simulink model "VCUHVACT"  (R2024b)
settings: Solver=FixedStepDiscrete  StartTime=0.0  StopTime=10.0  FixedStep=0.1  RelTol=1e-3
libraries: simulink x3
settings Model: Creator=32032  LastModifiedBy=32032
settings DataIOCC: SaveFormat=StructureWithTime
settings OptimizationCC: DefaultParameterBehavior=Inlined  EnhancedBackFolding=on  PassReuseOutputArgsAs=Individual arguments  ZeroExternalMemoryAtStartup=off  ZeroInternalMemoryAtStartup=off  OptimizeBlockOrder=speed  DifferentSizesBufferReuse=on  OptimizationCustomize=off  EfficientTunableParamExpr=on
settings DebuggingCC: ParameterTunabilityLossMsg=error
settings ModelReferenceCC: ModelReferenceNumInstancesAllowed=Single
settings SFSimCC: MATLABDynamicMemAlloc=off
settings RTWCC: Description=AUTOSAR  SystemTargetFile=autosar.tlc  GenCodeOnly=on  TemplateMakefile=ert_default_tmf  DataTypeReplacement=CDataTypesFixedWidth
settings CodeAppCC: ForceParamTrailComments=on  IgnoreCustomStorageClasses=off  OperatorAnnotations=on  SimulinkDataObjDesc=on  SFDataObjDesc=on  InsertBlockDesc=on
settings STFCustomTargetCC: TargetLangStandard=C99 (ISO)  MultiwordLength=256  ParMdlRefBuildCompliant=on  CompOptLevelCompliant=on  IncludeMdlTerminateFcn=off  CombineOutputUpdateFcns=on  SuppressErrorStatus=on  ERTCustomFileBanners=on  SupportNonFinite=off  SupportComplex=off  SupportContinuousTime=off  SupportNonInlinedSFcns=off  RemoveResetFunc=on  MATLABClassNameForMDSCustomization=Simulink.SoftwareTarget.ERTCustomization  AutosarCompliant=on  UseToolchainInfoCompliant=on  LookupTableObjectStructAxisOrder=2,1,3,4,...  LUTObjectStructOrderEvenSpacing=Size,Table,Breakpoints  SystemTargetFile=autosar.tlc
settings ERTTargetCC: TargetLangStandard=C99 (ISO)  ConcurrentExecutionCompliant=off  IncludeMdlTerminateFcn=off  SuppressErrorStatus=on  SupportNonFinite=off  SupportComplex=off  ModelStepFunctionPrototypeControlCompliant=off  CPPClassGenCompliant=off  AutosarCompliant=on  LookupTableObjectStructAxisOrder=2,1,3,4,...  LUTObjectStructOrderEvenSpacing=Size,Table,Breakpoints  ERTCustomFileTemplate=example_file_process.tlc  BooleanTrueId=TRUE  BooleanFalseId=FALSE

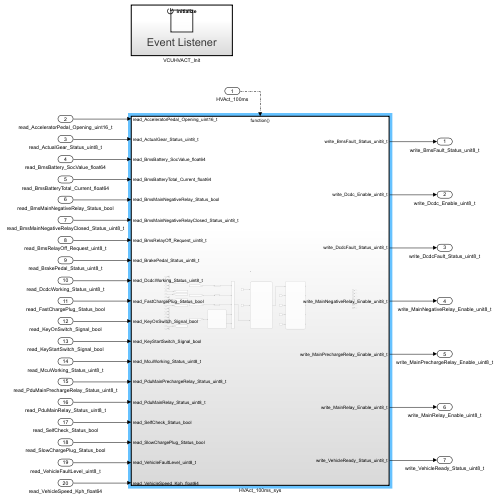
[thumbnail: Simulink's stored preview of the top-level diagram]
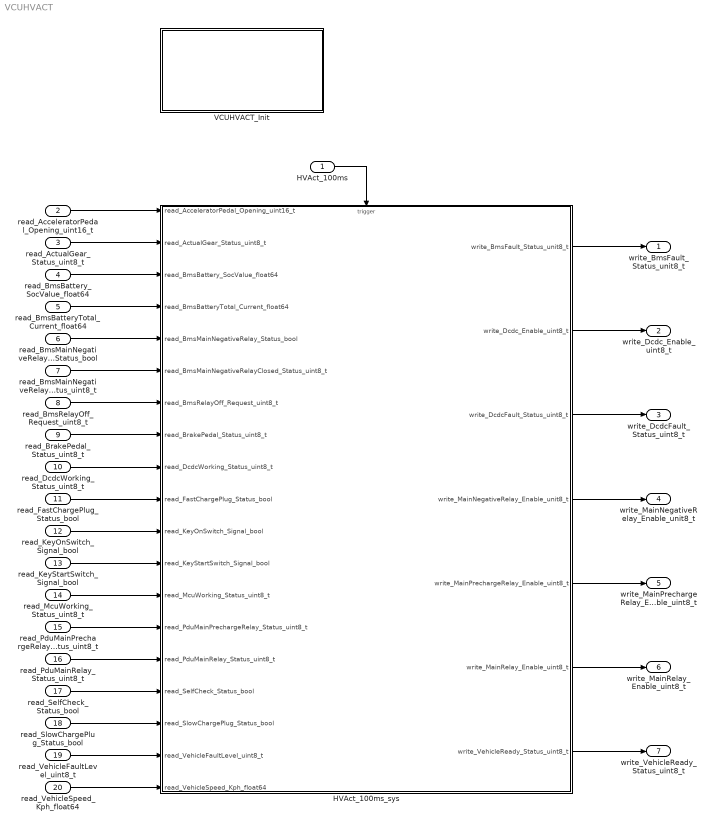
== system VCUHVACT ==
  HVAct_100ms : Inport  SampleTime=0.1  OutputFunctionCall=on
  read_AcceleratorPedal_Opening_uint16_t : Inport  Port=2  OutDataTypeStr=uint16  PortDimensions=1
  read_ActualGear_Status_uint8_t : Inport  Port=3  OutDataTypeStr=uint8  PortDimensions=1
  read_BmsBattery_SocValue_float64 : Inport  Port=4  OutDataTypeStr=double  PortDimensions=1
  read_BmsBatteryTotal_Current_float64 : Inport  Port=5  OutDataTypeStr=double  PortDimensions=1
  read_BmsMainNegativeRelay_Status_bool : Inport  Port=6  OutDataTypeStr=boolean  PortDimensions=1
  read_BmsMainNegativeRelayClosed_Status_uint8_t : Inport  Port=7  OutDataTypeStr=uint8  PortDimensions=1
  read_BmsRelayOff_Request_uint8_t : Inport  Port=8  OutDataTypeStr=uint8  PortDimensions=1
  read_BrakePedal_Status_uint8_t : Inport  Port=9  OutDataTypeStr=uint8  PortDimensions=1
  read_DcdcWorking_Status_uint8_t : Inport  Port=10  OutDataTypeStr=uint8  PortDimensions=1
  read_FastChargePlug_Status_bool : Inport  Port=11  OutDataTypeStr=boolean  PortDimensions=1
  read_KeyOnSwitch_Signal_bool : Inport  Port=12  OutDataTypeStr=boolean  PortDimensions=1
  read_KeyStartSwitch_Signal_bool : Inport  Port=13  OutDataTypeStr=boolean  PortDimensions=1
  read_McuWorking_Status_uint8_t : Inport  Port=14  OutDataTypeStr=uint8  PortDimensions=1
  read_PduMainPrechargeRelay_Status_uint8_t : Inport  Port=15  OutDataTypeStr=uint8  PortDimensions=1
  read_PduMainRelay_Status_uint8_t : Inport  Port=16  OutDataTypeStr=uint8  PortDimensions=1
  read_SelfCheck_Status_bool : Inport  Port=17  OutDataTypeStr=boolean  PortDimensions=1
  read_SlowChargePlug_Status_bool : Inport  Port=18  OutDataTypeStr=boolean  PortDimensions=1
  read_VehicleFaultLevel_uint8_t : Inport  Port=19  OutDataTypeStr=uint8  PortDimensions=1
  read_VehicleSpeed_Kph_float64 : Inport  Port=20  OutDataTypeStr=double  PortDimensions=1
  HVAct_100ms_sys : Subsystem
  VCUHVACT_Init : Subsystem
  write_BmsFault_Status_unit8_t : Outport  OutDataTypeStr=uint8  PortDimensions=1
  write_Dcdc_Enable_uint8_t : Outport  Port=2  OutDataTypeStr=uint8  PortDimensions=1
  write_DcdcFault_Status_uint8_t : Outport  Port=3  OutDataTypeStr=uint8  PortDimensions=1
  write_MainNegativeRelay_Enable_unit8_t : Outport  Port=4  OutDataTypeStr=uint8  PortDimensions=1
  write_MainPrechargeRelay_Enable_uint8_t : Outport  Port=5  OutDataTypeStr=uint8  PortDimensions=1
  write_MainRelay_Enable_uint8_t : Outport  Port=6  OutDataTypeStr=uint8  PortDimensions=1
  write_VehicleReady_Status_uint8_t : Outport  Port=7  OutDataTypeStr=uint8  PortDimensions=1
  wires:
  read_AcceleratorPedal_Opening_uint16_t/1 -> HVAct_100ms_sys/1(read_AcceleratorPedal_Opening_uint16_t)
  read_ActualGear_Status_uint8_t/1 -> HVAct_100ms_sys/2(read_ActualGear_Status_uint8_t)
  read_BmsBattery_SocValue_float64/1 -> HVAct_100ms_sys/3(read_BmsBattery_SocValue_float64)
  read_BmsBatteryTotal_Current_float64/1 -> HVAct_100ms_sys/4(read_BmsBatteryTotal_Current_float64)
  read_BmsMainNegativeRelay_Status_bool/1 -> HVAct_100ms_sys/5(read_BmsMainNegativeRelay_Status_bool)
  read_BmsMainNegativeRelayClosed_Status_uint8_t/1 -> HVAct_100ms_sys/6(read_BmsMainNegativeRelayClosed_Status_uint8_t)
  read_BmsRelayOff_Request_uint8_t/1 -> HVAct_100ms_sys/7(read_BmsRelayOff_Request_uint8_t)
  read_BrakePedal_Status_uint8_t/1 -> HVAct_100ms_sys/8(read_BrakePedal_Status_uint8_t)
  read_DcdcWorking_Status_uint8_t/1 -> HVAct_100ms_sys/9(read_DcdcWorking_Status_uint8_t)
  read_FastChargePlug_Status_bool/1 -> HVAct_100ms_sys/10(read_FastChargePlug_Status_bool)
  read_KeyOnSwitch_Signal_bool/1 -> HVAct_100ms_sys/11(read_KeyOnSwitch_Signal_bool)
  read_KeyStartSwitch_Signal_bool/1 -> HVAct_100ms_sys/12(read_KeyStartSwitch_Signal_bool)
  read_McuWorking_Status_uint8_t/1 -> HVAct_100ms_sys/13(read_McuWorking_Status_uint8_t)
  read_PduMainPrechargeRelay_Status_uint8_t/1 -> HVAct_100ms_sys/14(read_PduMainPrechargeRelay_Status_uint8_t)
  read_PduMainRelay_Status_uint8_t/1 -> HVAct_100ms_sys/15(read_PduMainRelay_Status_uint8_t)
  read_SelfCheck_Status_bool/1 -> HVAct_100ms_sys/16(read_SelfCheck_Status_bool)
  read_SlowChargePlug_Status_bool/1 -> HVAct_100ms_sys/17(read_SlowChargePlug_Status_bool)
  read_VehicleFaultLevel_uint8_t/1 -> HVAct_100ms_sys/18(read_VehicleFaultLevel_uint8_t)
  read_VehicleSpeed_Kph_float64/1 -> HVAct_100ms_sys/19(read_VehicleSpeed_Kph_float64)
  HVAct_100ms_sys/1(write_BmsFault_Status_unit8_t) -> write_BmsFault_Status_unit8_t/1
  HVAct_100ms_sys/2(write_Dcdc_Enable_uint8_t) -> write_Dcdc_Enable_uint8_t/1
  HVAct_100ms_sys/3(write_DcdcFault_Status_uint8_t) -> write_DcdcFault_Status_uint8_t/1
  HVAct_100ms_sys/4(write_MainNegativeRelay_Enable_unit8_t) -> write_MainNegativeRelay_Enable_unit8_t/1
  HVAct_100ms_sys/5(write_MainPrechargeRelay_Enable_uint8_t) -> write_MainPrechargeRelay_Enable_uint8_t/1
  HVAct_100ms_sys/6(write_MainRelay_Enable_uint8_t) -> write_MainRelay_Enable_uint8_t/1
  HVAct_100ms_sys/7(write_VehicleReady_Status_uint8_t) -> write_VehicleReady_Status_uint8_t/1
  HVAct_100ms/1 -> HVAct_100ms_sys/Trigger

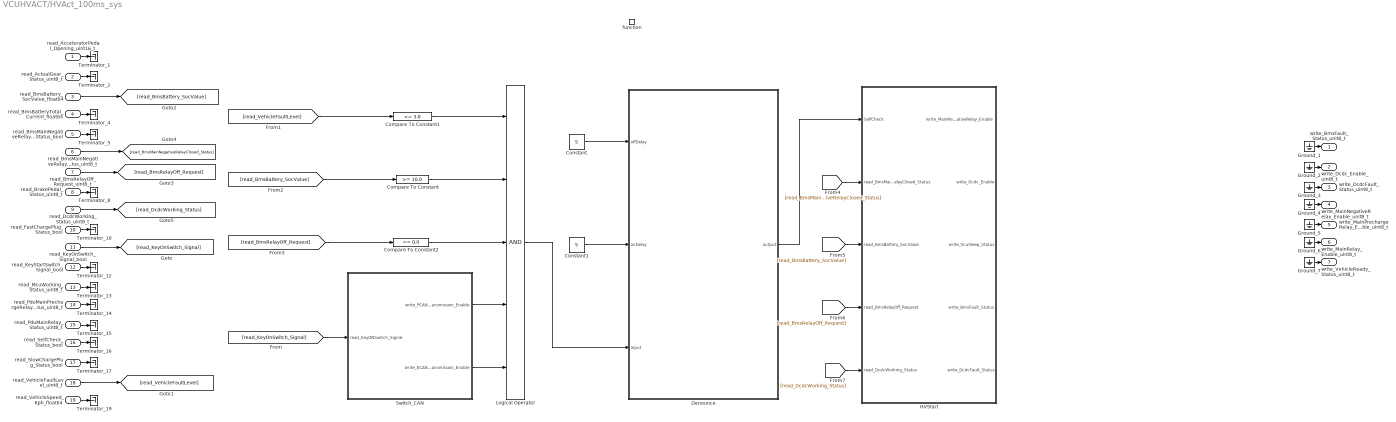
== system VCUHVACT/HVAct_100ms_sys ==
  read_AcceleratorPedal_Opening_uint16_t : Inport
  read_ActualGear_Status_uint8_t : Inport  Port=2
  read_BmsBattery_SocValue_float64 : Inport  Port=3
  read_BmsBatteryTotal_Current_float64 : Inport  Port=4
  read_BmsMainNegativeRelay_Status_bool : Inport  Port=5
  read_BmsMainNegativeRelayClosed_Status_uint8_t : Inport  Port=6
  read_BmsRelayOff_Request_uint8_t : Inport  Port=7
  read_BrakePedal_Status_uint8_t : Inport  Port=8
  read_DcdcWorking_Status_uint8_t : Inport  Port=9
  read_FastChargePlug_Status_bool : Inport  Port=10
  read_KeyOnSwitch_Signal_bool : Inport  Port=11
  read_KeyStartSwitch_Signal_bool : Inport  Port=12
  read_McuWorking_Status_uint8_t : Inport  Port=13
  read_PduMainPrechargeRelay_Status_uint8_t : Inport  Port=14
  read_PduMainRelay_Status_uint8_t : Inport  Port=15
  read_SelfCheck_Status_bool : Inport  Port=16
  read_SlowChargePlug_Status_bool : Inport  Port=17
  read_VehicleFaultLevel_uint8_t : Inport  Port=18
  read_VehicleSpeed_Kph_float64 : Inport  Port=19
  function : TriggerPort  TriggerType=function-call  VariantControl=(inherit)  SampleTimeType=periodic  SampleTime=-1
  Compare To Constant : simulink/Logic and Bit Operations/Compare To Constant  relop=>=  const=10.0  OutDataTypeStr=boolean
  Compare To Constant1 : simulink/Logic and Bit Operations/Compare To Constant  relop=<=  const=3.0  OutDataTypeStr=boolean
  Compare To Constant2 : simulink/Logic and Bit Operations/Compare To Constant  relop===  const=0.0  OutDataTypeStr=boolean
  Constant : Constant  Value=5
  Constant1 : Constant  Value=5
  Denounce : Stateflow chart  TreatAsAtomicUnit=on
  Ground_{1..7} (7 alike) : Ground
  HVStart : Stateflow chart  TreatAsAtomicUnit=on
  Logical Operator : Logic  Inputs=5  AllPortsSameDT=off  OutDataTypeStr=boolean
  Switch_CAN : Stateflow chart  TreatAsAtomicUnit=on
  Terminator_{1..2,4..5,8,10,12..17,19} (13 alike) : Terminator
  write_BmsFault_Status_unit8_t : Outport
      settings: EnsureOutportIsVirtual=on
  write_Dcdc_Enable_uint8_t : Outport  Port=2
      settings: EnsureOutportIsVirtual=on
  write_DcdcFault_Status_uint8_t : Outport  Port=3
      settings: EnsureOutportIsVirtual=on
  write_MainNegativeRelay_Enable_unit8_t : Outport  Port=4
      settings: EnsureOutportIsVirtual=on
  write_MainPrechargeRelay_Enable_uint8_t : Outport  Port=5
      settings: EnsureOutportIsVirtual=on
  write_MainRelay_Enable_uint8_t : Outport  Port=6
      settings: EnsureOutportIsVirtual=on
  write_VehicleReady_Status_uint8_t : Outport  Port=7
      settings: EnsureOutportIsVirtual=on
  wires:
  read_AcceleratorPedal_Opening_uint16_t/1 -> Terminator_1/1
  read_ActualGear_Status_uint8_t/1 -> Terminator_2/1
  read_BmsBattery_SocValue_float64/1 -> [read_BmsBattery_SocValue]
  read_BmsBatteryTotal_Current_float64/1 -> Terminator_4/1
  read_BmsMainNegativeRelay_Status_bool/1 -> Terminator_5/1
  read_BmsMainNegativeRelayClosed_Status_uint8_t/1 -> [read_BmsMainNegativeRelayClosed_Status]
  read_BmsRelayOff_Request_uint8_t/1 -> [read_BmsRelayOff_Request]
  read_BrakePedal_Status_uint8_t/1 -> Terminator_8/1
  read_DcdcWorking_Status_uint8_t/1 -> [read_DcdcWorking_Status]
  read_FastChargePlug_Status_bool/1 -> Terminator_10/1
  read_KeyOnSwitch_Signal_bool/1 -> [read_KeyOnSwitch_Signal]
  read_KeyStartSwitch_Signal_bool/1 -> Terminator_12/1
  read_McuWorking_Status_uint8_t/1 -> Terminator_13/1
  read_PduMainPrechargeRelay_Status_uint8_t/1 -> Terminator_14/1
  read_PduMainRelay_Status_uint8_t/1 -> Terminator_15/1
  read_SelfCheck_Status_bool/1 -> Terminator_16/1
  read_SlowChargePlug_Status_bool/1 -> Terminator_17/1
  read_VehicleFaultLevel_uint8_t/1 -> [read_VehicleFaultLevel]
  read_VehicleSpeed_Kph_float64/1 -> Terminator_19/1
  Ground_1/1 -> write_BmsFault_Status_unit8_t/1
  Ground_2/1 -> write_Dcdc_Enable_uint8_t/1
  Ground_3/1 -> write_DcdcFault_Status_uint8_t/1
  Ground_4/1 -> write_MainNegativeRelay_Enable_unit8_t/1
  Ground_5/1 -> write_MainPrechargeRelay_Enable_uint8_t/1
  Ground_6/1 -> write_MainRelay_Enable_uint8_t/1
  Ground_7/1 -> write_VehicleReady_Status_uint8_t/1
  [read_KeyOnSwitch_Signal] -> Switch_CAN/1(read_KeyONSwitch_Signal)
  [read_BmsBattery_SocValue] -> Compare To Constant/1
  [read_VehicleFaultLevel] -> Compare To Constant1/1
  [read_BmsRelayOff_Request] -> Compare To Constant2/1
  Compare To Constant/1 -> Logical Operator/2
  Compare To Constant1/1 -> Logical Operator/1
  Compare To Constant2/1 -> Logical Operator/3
  Switch_CAN/2(write_ECANTransmission_Enable) -> Logical Operator/5
  Switch_CAN/1(write_PCANTransmission_Enable) -> Logical Operator/4
  Logical Operator/1 -> Denounce/3(input)
  Constant/1 -> Denounce/1(offDelay)
  Constant1/1 -> Denounce/2(onDelay)
  Denounce/1(output) -> HVStart/1(SelfCheck)
  [read_BmsMainNegativeRelayClosed_Status] -> HVStart/2(read_BmsMainNegativeRelayClosed_Status)
  [read_BmsBattery_SocValue] -> HVStart/3(read_BmsBattery_SocValue)
  [read_BmsRelayOff_Request] -> HVStart/4(read_BmsRelayOff_Request)
  [read_DcdcWorking_Status] -> HVStart/5(read_DcdcWorking_Status)

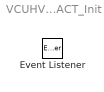
== system VCUHVACT/VCUHVACT_Init ==
  Event Listener : EventListener  EventName=reset

== stateflow chart VCUHVACT/HVAct_100ms_sys/Switch_CAN ==
  state Init
    write_PCANTransmission_Enable=false;
    write_ECANTransmission_Enable=false;
  state On
    write_PCANTransmission_Enable=true;
    write_ECANTransmission_Enable=true;
  (default) -> Init
  On -> Init : [read_KeyONSwitch_Signal~=1]
  Init -> On : [read_KeyONSwitch_Signal==1]
  data: read_KeyONSwitch_Signal input; write_PCANTransmission_Enable output boolean; write_ECANTransmission_Enable output boolean

== stateflow chart VCUHVACT/HVAct_100ms_sys/Denounce ==
  (default) -> (junction 6)
  (junction 5) -> (junction 1) : {counter2 = counter2 + 1;counter1=0;}
  (junction 6) -> (junction 5) [order 1] : [input==0]
  (junction 6) -> (junction 18) [order 2] : [input==1]
  (junction 18) -> (junction 19) : {counter1 = counter1 + 1;counter2=0;}
  (junction 1) -> (junction 12) [order 2]
  (junction 19) -> (junction 12) [order 2]
  (junction 1) -> (junction 13) [order 1] : [counter2>offDelay]
  (junction 19) -> (junction 11) [order 1] : [counter1>onDelay]
  (junction 13) -> (junction 12) : {output=0;counter2=offDelay;}
  (junction 11) -> (junction 12) : {output=1;counter1=onDelay;}
  data: offDelay input; onDelay input; output output =0; counter1 local =0; counter2 local =0; input input

== stateflow chart VCUHVACT/HVAct_100ms_sys/HVStart ==
  state Init
    en:
    write_VcuSleep_Status=0;
    write_MainNegativeRelay_Enable=0;
    write_Dcdc_Enable=0;
    counter=0;
    du:
    counter=counter+1;
  state HV_On
    state HV_ON1
      en:
      write_MainNegativeRelay_Enable=1;
      counter=0;
      du:
      counter=counter+1;
    state HV_ON2
      en:
      counter=0;
      du:
      counter=counter+1;
    state HV_ON3
      en:
      write_Dcdc_Enable=1;
      counter=0;
      du:
      counter=counter+1;
    (default) -> HV_ON1
    HV_ON1 -> HV_ON2 [order 2] : [read_BmsMainNegativeRelayClosed_Status==1]
    HV_ON2 -> HV_ON3 : [counter>=30]
  state HV_OFFStandy
    state HV_OFF2
      en:
      write_MainNegativeRelay_Enable=1;
      counter=0;
      du:
      counter=counter+1;
    state HV_OFF1
      en:
      write_Dcdc_Enable=0;
      counter=0;
      du:
      counter=counter+1;
    HV_OFF1 -> HV_OFF2 : [counter>=30||read_BmsBattery_SocValue<10]
    (default) -> HV_OFF1
  state HV_OFF
    en:
    counter=0;
    du:
    counter=counter+1;
  state HV_Standy
  (default) -> Init
  (junction 36) -> Init
  HV_OFF2 -> (junction 36) [order 2] : [read_BmsRelayOff_Request==1&&SelfCheck~=1]
  (junction 40) -> Init
  HV_OFF2 -> (junction 40) [order 1] : [counter>=30]{write_BmsFault_Status=1}
  Init -> HV_On : [counter>=30&&SelfCheck==1]
  HV_ON1 -> HV_OFF2 [order 1] : [counter>=30]
  HV_On -> HV_OFFStandy : [SelfCheck~=1]
  HV_OFF -> HV_OFFStandy [order 2] : [counter>=30]
  HV_ON3 -> HV_Standy [order 1] : [read_DcdcWorking_Status==1]
  HV_ON3 -> HV_Standy [order 2] : [counter>=30]{write_DcdcFault_Status=1}
  HV_OFF -> HV_Standy [order 1] : [SelfCheck==1]
  HV_Standy -> HV_OFF : [SelfCheck~=1]
  data: counter local; SelfCheck input; write_MainNegativeRelay_Enable output; write_Dcdc_Enable output; write_VcuSleep_Status output; read_BmsMainNegativeRelayClosed_Status input; read_BmsBattery_SocValue input; read_BmsRelayOff_Request input; read_DcdcWorking_Status input; write_BmsFault_Status output; write_DcdcFault_Status output
